simulink model "Maglev_simulation_new"  (Simulink 8.7)
settings: Solver=VariableStepAuto  SolverMode=SingleTasking  StartTime=0.0  StopTime=10  FixedStep=0.0001  MaxStep=1e-3  RelTol=1e-4
values from neighbouring files (symbols this model uses):
  g = model.g    [Levitation.m]
  K = lqr(sys,eye(3),1,zeros(3,1))    [Levitation.m]
  ki = 2.8964    [Levitation.m]
  m = model.m    [Levitation.m]
  u0 = (x0(3)-uc)/ki    [Levitation.m]
  x0 = zeros(3,1)    [Levitation.m]
undefined symbols (not defined in the file): Par_Fem, uc
libraries: simulink x1
settings Model: Creator=Kamil  LastModifiedBy=Marcin
settings DataIOCC: SaveFormat=Dataset  SaveOutput=off  SaveTime=off
settings OptimizationCC: ExpressionDepthLimit=2147483647  LifeSpan=1
settings DebuggingCC: FcnCallInpInsideContextMsg=EnableAllAsWarning  StateNameClashWarn=warning
settings HardwareCC: ProdBitPerPointer=64  ProdLargestAtomicFloat=Float  ProdIntDivRoundTo=Zero  ProdEndianess=LittleEndian  ProdHWDeviceType=Specified
settings ModelReferenceCC: PropagateSignalLabelsOutOfModel=on
settings GRTTargetCC: CombineOutputUpdateFcns=off  GRTInterface=on
settings ConfigComp: CovModelRefEnable=off

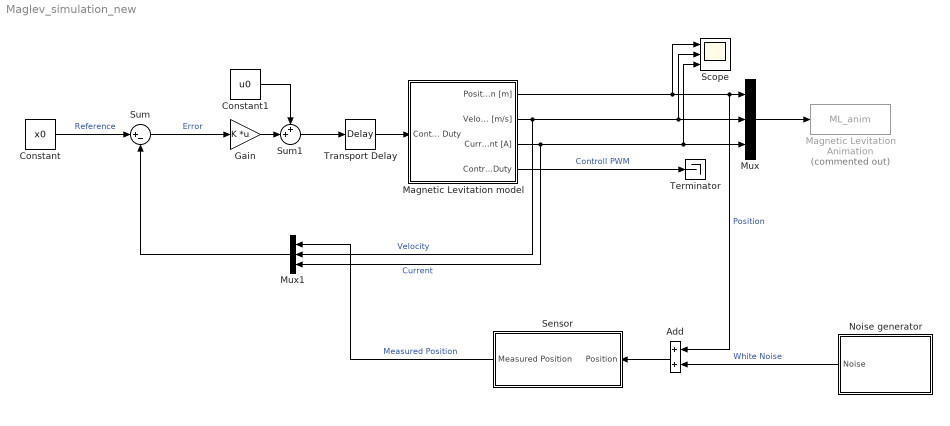
== system Maglev_simulation_new ==
  Add : Sum
  Constant : Constant  Value=x0
  Constant1 : Constant  Value=u0
  Gain : Gain  Gain=K  Multiplication=Matrix(K*u)
  Magnetic Levitation Animation : S-Function  Commented=on  FunctionName=ML_anim  Parameters=0.01  SFunctionDeploymentMode=off  EnableBusSupport=off
      settings: DeleteFcn=if ~isempty(findobj('type','figure','name','onecart Animation'));close('onecart Animation'); end;
  Magnetic Levitation model : Subsystem  mask(Magnetic levitation - model){x0=x0, m=m, g=g, Par_Fem=Par_Fem, Par_ActStat=[ki, uc], Par_ActDyn=[1.4142e-4, 4.5626e-3], Cnstr=[0, 1, 0.03884, 2.38]}
      mask prompts: x0 "Initial state (position [m], velocity [m/s], current [A]):"; m "Ball mass [kg]"; g "Gravity constant [m/s2]"; Par_Fem "EM Forceparametrs (FemP1 [H], FemP2 [m]):"; Par_ActStat "Actuator parameters (ki [A], ci[A]):"; Par_ActDyn "Actuator parameters fi (fiP1 [m*s], fiP2 [m]):"; Cnstr "Constraints (umin, umax, x3min, x3max):"
      mask help:
      | Nonlinear model of the Magnetic Levitation
      | INTECO (c)
      mask init:
      | ki = Par_ActStat(1);
      | ci = Par_ActStat(2);
      | P1i = Par_ActDyn(1);
      | P2i = Par_ActDyn(2);
      | umin = Cnstr(1);
      | umax = Cnstr(2);
      | x3min = Cnstr(3);
      | x3max = Cnstr(4);
      mask Display:
      | plot(0,0,100,100,[15,5,5,18,82,95,95,85,85,95],[5,5,95,95,95,95,5,5,15,15], [5,15,15,15,25,75,85,85],[15, 15, 5,85,85,85,85,5 ], [50,44,44,38,38,35,35,65,65,62,62,56,56,50],[70,70,81,81,70,70,84,84,70,70,81,81,70,70], [50.00, 50.80, 51.59, 52.36, 53.12, 53.84, 54.52, 55.15, 55.74, 56.27, 56.73, 57.13, 57.46, 57.71, 57.88, 57.98, 58.00, 57.93, 57.79, 57.57, 57.27, 56.91, 56.47, 55.97, 55.40, 54.79, 54.12, 53.42, 52.68, 51.91, 51.13, 50.33, 49.53, 48.74, 47.96, 47.19, 46.46, 45.76, 45.11, 44.50, 43.95, 43.45, 43.03, 42.67, 42.39, 42.18, 42.05, 42.00, 42.03, 42.14, 42.33, 42.59, 42.93, 43.34, 43.82, 44.36, 44.95, 45.59, 46.28, 47.01, 47.76, 48.54, 49.34, ], [58.00, 57.96, 57.84, 57.64, 57.37, 57.02, 56.60, 56.12, 55.57, 54.97, 54.32, 53.63, 52.90, 52.14, 51.36, 50.57, 49.77, 48.97, 48.18, 47.41, 46.67, 45.96, 45.29, 44.67, 44.10, 43.59, 43.14, 42.77, 42.46, 42.23, 42.08, 42.01, 42.01, 42.10, 42.27, 42.51, 42.83, 43.22, 43.67, 44.19, 44.77, 45.40, 46.08, 46.79, 47.54, 48.31, 49.10, 49.90, 50.70, 51.49, 52.27, 53.02, 53.75, 54.43, 55.08, 55.67, 56.20, 56.68, 57.08, 57.42, 57.68, 57.87, 57.97, ],  [15,15,15,85,85,15],[22,28,28,28,22,22])
      | fprintf('\n\n\n\n\nMagLev');
  Mux : Mux  Inputs=3
  Mux1 : Mux  Inputs=3
  Noise generator : Subsystem
  Scope : Scope  NumInputPorts=3
  Sensor : Subsystem
  Sum : Sum  Inputs=|+-
  Sum1 : Sum  Inputs=++|
  Terminator : Terminator
  Transport Delay : TransportDelay  DelayTime=1e-3  InitialOutput=u0
  wires:
  Magnetic Levitation model/1(Position [m]) -> Scope/1, Mux/1, Add/1  "Position"
  Noise generator/1(Noise) -> Add/2  "White Noise"
  Add/1 -> Sensor/1(Position)
  Magnetic Levitation model/2(Velocity [m/s]) -> Mux1/2, Scope/2, Mux/2  "Velocity"
  Magnetic Levitation model/3(Current [A]) -> Mux1/3, Scope/3, Mux/3  "Current"
  Magnetic Levitation model/4(Control PWMDuty) -> Terminator/1  "Controll PWM"
  Mux/1 -> Magnetic Levitation Animation/1
  Sensor/1(Measured Position) -> Mux1/1  "Measured Position"
  Transport Delay/1 -> Magnetic Levitation model/1(Control  - PWM Duty)
  Constant/1 -> Sum/1  "Reference"
  Mux1/1 -> Sum/2
  Sum/1 -> Gain/1  "Error"
  Gain/1 -> Sum1/2
  Sum1/1 -> Transport Delay/1
  Constant1/1 -> Sum1/1

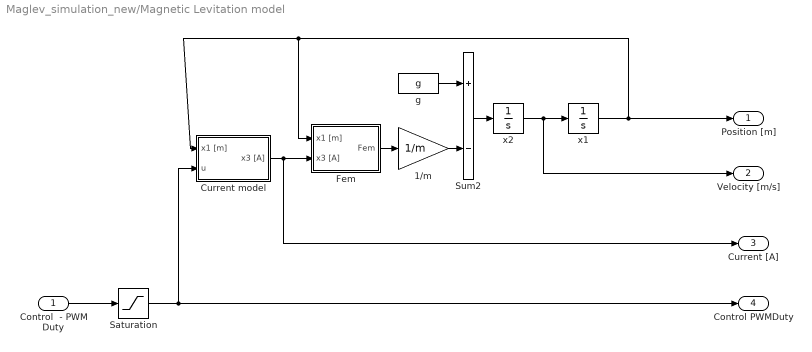
== system Maglev_simulation_new/Magnetic Levitation model ==
  Control  - PWM Duty : Inport
  1/m : Gain  Gain=1/m  SaturateOnIntegerOverflow=on  OutDataTypeStr=Inherit: Same as input  ParamDataTypeStr=Inherit: Same as input
  Current model : Subsystem
  Fem : Subsystem  mask{FemP1=Par_Fem(1), FemP2=Par_Fem(2)}
  Saturation : Saturate  UpperLimit=umax  LowerLimit=umin
  Sum2 : Sum  Inputs=+-  SaturateOnIntegerOverflow=on  InputSameDT=on  OutDataTypeStr=Inherit: Same as first input
  g : Constant  Value=g
  x1 : Integrator  InitialCondition=x0(1)  LimitOutput=on  UpperSaturationLimit=0.02  LowerSaturationLimit=0.0001
  x2 : Integrator  InitialCondition=x0(2)  UpperSaturationLimit=10  LowerSaturationLimit=-10
  Position [m] : Outport  InitialOutput=0
  Velocity [m/s] : Outport  Port=2  InitialOutput=0
  Current [A] : Outport  Port=3  InitialOutput=0
  Control PWMDuty : Outport  Port=4  InitialOutput=0
  wires:
  Current model/1(x3 [A]) -> Current [A]/1, Fem/2(x3 [A])
  x1/1 -> Position [m]/1, Fem/1(x1 [m]), Current model/1(x1 [m])
  1/m/1 -> Sum2/2
  Fem/1(Fem) -> 1/m/1
  Sum2/1 -> x2/1
  g/1 -> Sum2/1
  x2/1 -> Velocity [m/s]/1, x1/1
  Saturation/1 -> Current model/2(u), Control PWMDuty/1
  Control  - PWM Duty/1 -> Saturation/1

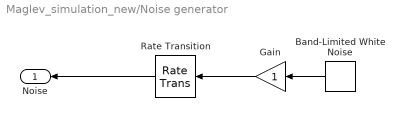
== system Maglev_simulation_new/Noise generator ==
  Band-Limited White Noise : simulink/Sources/Band-Limited White Noise  Cov=[1e-12]  Ts=0.01  seed=[floor(rand*100)]
  Gain : Gain
  Rate Transition : RateTransition
  Noise : Outport
  wires:
  Rate Transition/1 -> Noise/1
  Band-Limited White Noise/1 -> Gain/1
  Gain/1 -> Rate Transition/1

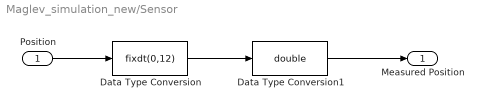
== system Maglev_simulation_new/Sensor ==
  Position : Inport
  Data Type Conversion : DataTypeConversion  OutMin=[0]  OutMax=[0.02]  OutDataTypeStr=fixdt(0,12)
  Data Type Conversion1 : DataTypeConversion  OutMin=[0]  OutMax=[2]  OutDataTypeStr=double
  Measured Position : Outport
  wires:
  Data Type Conversion1/1 -> Measured Position/1
  Data Type Conversion/1 -> Data Type Conversion1/1
  Position/1 -> Data Type Conversion/1

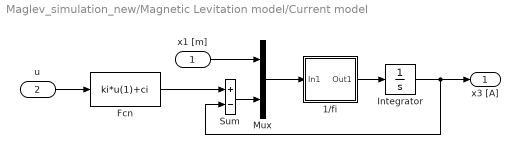
== system Maglev_simulation_new/Magnetic Levitation model/Current model ==
  x1 [m] : Inport
  u : Inport  Port=2
  1/fi : Subsystem  mask(Current function fi){P1=P1i, P2=P2i}
      mask prompts: P1 "fiP1 [H]:"; P2 "fiP2 [m]:"
      mask Display: plot([0    0.0010    0.0020    0.0030    0.0040    0.0050    0.0060    0.0070   0.0080    0.0090    0.0100    0.0110    0.0120    0.0130    0.0140    0.0150], 1./[0.0292    0.0284    0.0277    0.0271    0.0266    0.0262    0.0258    0.0255    0.0252    0.0250    0.0248    0.0246    0.0245    0.0243    0.0242    0.0241]);
  Fcn : Fcn  Expr=ki*u(1)+ci
  Integrator : Integrator  InitialCondition=x0(3)  LimitOutput=on  UpperSaturationLimit=x3max  LowerSaturationLimit=x3min
  Mux : Mux  Inputs=2
  Sum : Sum  Inputs=+-  SaturateOnIntegerOverflow=on  InputSameDT=on  OutDataTypeStr=Inherit: Same as first input
  x3 [A] : Outport
  wires:
  x1 [m]/1 -> Mux/1
  Mux/1 -> 1/fi/1(In1)
  Sum/1 -> Mux/2
  Fcn/1 -> Sum/1
  Integrator/1 -> Sum/2, x3 [A]/1
  1/fi/1(Out1) -> Integrator/1
  u/1 -> Fcn/1

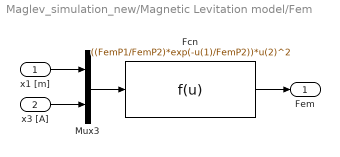
== system Maglev_simulation_new/Magnetic Levitation model/Fem ==
  x1 [m] : Inport
  x3 [A] : Inport  Port=2
  Fcn : Fcn  Expr=((FemP1/FemP2)*exp(-u(1)/FemP2))*u(2)^2
  Mux3 : Mux  Inputs=2
  Fem : Outport
  wires:
  Mux3/1 -> Fcn/1
  x3 [A]/1 -> Mux3/2
  x1 [m]/1 -> Mux3/1
  Fcn/1 -> Fem/1

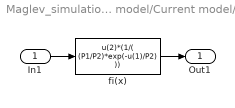
== system Maglev_simulation_new/Magnetic Levitation model/Current model/1/fi ==
  In1 : Inport
  fi(x) : Fcn  Expr=u(2)*(1/( (P1/P2)*exp(-u(1)/P2) ))
  Out1 : Outport
  wires:
  In1/1 -> fi(x)/1
  fi(x)/1 -> Out1/1
